simulink model "sl_RobotReal_RRR"  (R2018a)
settings: Solver=ode45  StartTime=0.0  StopTime=30  MaxStep=1e-3  RelTol=1e-3  EnableMultiTasking=on
values from neighbouring files (symbols this model uses):
  Aa_1 = Aa_1/50    (= 0.004)    [DatosSimAcDir_Exp.m]    (also in DatosSimSenoides.m = 1; DatosSimSenoides_Exp.m = 2)
  Aa_2 = Aa_2/30    (= 6.66666666667)    [DatosSimAcDir_Exp.m]    (also in DatosSimSenoides.m = 1; DatosSimSenoides_Exp.m = 0.5)
  Aa_3 = Aa_3/15    (= 0.266666666667)    [DatosSimAcDir_Exp.m]    (also in DatosSimSenoides.m = 5; DatosSimSenoides_Exp.m = 0.5)
  Ab_1 = Ab_1/50    (= 6e-05)    [DatosSimAcDir_Exp.m]    (also in DatosSimSenoides.m = 2; DatosSimSenoides_Exp.m = 3)
  Ab_3 = Ab_3/15    (= 1)    [DatosSimAcDir_Exp.m]    (also in DatosSimSenoides.m = 6; DatosSimSenoides_Exp.m = 2)
  Im_cc1 = Im_cc1/50    (= 0)    [DatosSimAcDir_Exp.m]    (also in DatosSimSenoides.m; DatosSimSenoides_Exp.m)
  Im_cc2 = Im_cc2/30    (= 96.6666666667)    [DatosSimAcDir_Exp.m]    (also in DatosSimSenoides.m = 0; DatosSimSenoides_Exp.m = 14)
  Im_cc3 = Im_cc3/15    (= 1)    [DatosSimAcDir_Exp.m]    (also in DatosSimSenoides.m = 0; DatosSimSenoides_Exp.m = 3)
  R1 = 50    [AnalisisFrecuencial.m]    (also in ComparativaModelo.m; DinamicaNE_RRR.m = R1; IdentificacParamDinam.m; Modelado_Dinamico_Gs.m = 1)
  R2 = 30    [AnalisisFrecuencial.m]    (also in ComparativaModelo.m; DinamicaNE_RRR.m = R2; IdentificacParamDinam.m; Modelado_Dinamico_Gs.m = 1)
  R3 = 15    [AnalisisFrecuencial.m]    (also in ComparativaModelo.m; DinamicaNE_RRR.m = R3; IdentificacParamDinam.m; Modelado_Dinamico_Gs.m = 1)
  tau1 = 1    [DatosSimAcDir_Exp.m]    (also in DatosSimSenoides.m = 5; DatosSimSenoides_Exp.m = 0.01)
  tau2 = 100    [DatosSimAcDir_Exp.m]    (also in DatosSimSenoides.m = 5; DatosSimSenoides_Exp.m = 1)
  tau3 = 20    [DatosSimAcDir_Exp.m]    (also in DatosSimSenoides.m = 5; DatosSimSenoides_Exp.m = 0.01)
  Tm = 0.001    [AnalisisFrecuencial.m]    (also in ComparativaModelo.m; DatosSimSenoides.m = 0.01; GDT_C_RRR.m; controlador.m)
  wa_1 = 10    [DatosSimAcDir_Exp.m]    (also in DatosSimSenoides.m = 0.5; DatosSimSenoides_Exp.m)
  wa_2 = 40    [DatosSimAcDir_Exp.m]    (also in DatosSimSenoides.m = 3; DatosSimSenoides_Exp.m = 15)
  wa_3 = 8    [DatosSimAcDir_Exp.m]    (also in DatosSimSenoides.m = 0.5; DatosSimSenoides_Exp.m)
  wb_1 = 3    [DatosSimAcDir_Exp.m]    (also in DatosSimSenoides.m = 1; DatosSimSenoides_Exp.m)
  wb_3 = 50    [DatosSimAcDir_Exp.m]    (also in DatosSimSenoides.m = 1; DatosSimSenoides_Exp.m = 3)
settings Model: ExtModeTrigMode=oneshot  ExtModeArmWhenConnect=off  Creator=mortega  LastModifiedBy=MAMG
settings DataIOCC: SaveFormat=Array  SignalLoggingSaveFormat=ModelDataLogs
settings OptimizationCC: BlockReduction=off  BooleanDataType=off  ExpressionDepthLimit=2147483647  InitFltsAndDblsToZero=on  LifeSpan=inf
settings DebuggingCC: SaveWithParameterizedLinksMsg=none  UnderspecifiedInitializationDetection=Classic  MergeDetectMultiDrivingBlocksExec=none  SignalResolutionControl=TryResolveAllWithWarning  MultiTaskDSMMsg=warning  MultiTaskCondExecSysMsg=none  FcnCallInpInsideContextMsg=warning  StateNameClashWarn=warning  SFUnexpectedBacktrackingDiag=warning  SFNoUnconditionalDefaultTransitionDiag=warning  SFExecutionAtInitializationDiag=none
settings HardwareCC: ProdBitPerPointer=32  ProdBitPerSizeT=32  ProdBitPerPtrDiffT=32  ProdLargestAtomicFloat=None  ProdIntDivRoundTo=Undefined  ProdEndianess=Unspecified  ProdWordSize=32  ProdHWDeviceType=32-bit Generic  TargetUnknown=on
settings ModelReferenceCC: PropagateSignalLabelsOutOfModel=off
settings CodeAppCC: StateflowObjectComments=on
settings GRTTargetCC: TargetFcnLib=ansi_tfl_tmw.mat  TargetLangStandard=C89/C90 (ANSI)  CombineOutputUpdateFcns=off  GRTInterface=on
settings ConfigComp: CovMetricSettings=dw  CovHtmlReporting=on  CovSaveCumulativeToWorkspaceVar=on  CovSaveSingleToWorkspaceVar=on  CovExternalEMLEnable=off

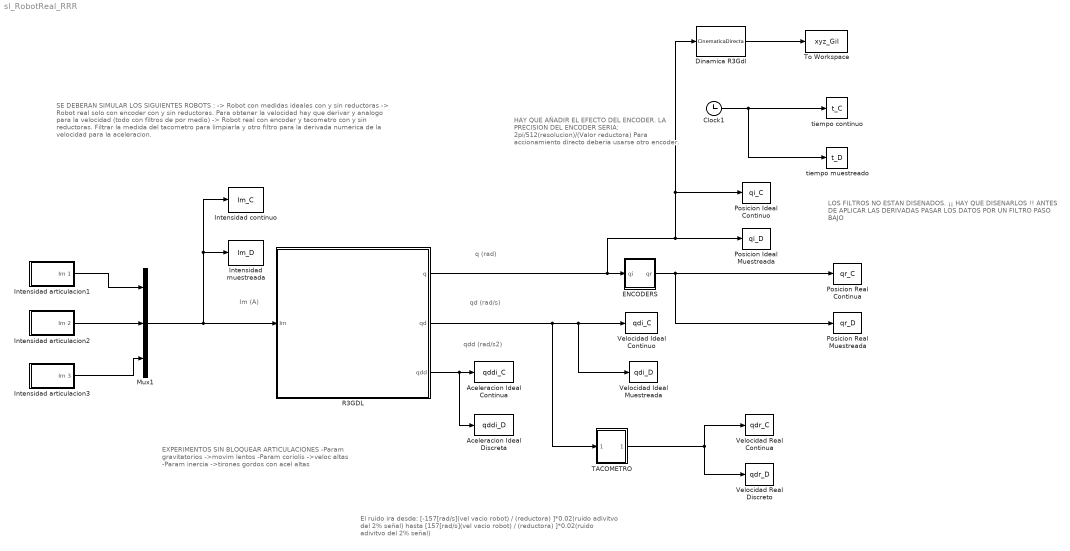
== system sl_RobotReal_RRR ==
  note: LOS FILTROS NO ESTAN DISENADOS.
      | ¡¡ HAY QUE DISENARLOS !!
      |
      | ANTES DE APLICAR LAS DERIVADAS PASAR
      | LOS DATOS POR UN FILTRO PASO BAJO
  note: SE DEBERAN SIMULAR LOS SIGUIENTES ROBOTS :
      | -> Robot con medidas ideales con y sin reductoras
      | -> Robot real solo con encoder con y sin reductoras. Para obtener la velocidad hay que derivar
      | y analogo para la velocidad
      | (todo con filtros de por medio)
      | -> Robot real con encoder y tacometro con y sin reductoras. Filtrar la medida del tacometro para limpiarla
      | y otro filtro para la derivada numerica de la
      | velocidad para la aceleracion.
  note: EXPERIMENTOS SIN BLOQUEAR ARTICULACIONES
      | -Param gravitatorios ->movim lentos
      | -Param coriolis ->veloc altas
      | -Param inercia ->tirones gordos con acel altas
  note: El ruido ira desde:
      | [-157[rad/s](vel vacio robot) / (reductora) ]*0.02(ruido adivitvo del 2% señal)
      | hasta
      | [157[rad/s](vel vacio robot) / (reductora) ]*0.02(ruido adivitvo del 2% señal)
  note: HAY QUE AÑADIR EL EFECTO DEL ENCODER.
      | LA PRECISION DEL ENCODER SERIA:
      | 2pi/512(resolucion)/(Valor reductora)
      |
      | Para accionamiento directo deberia usarse otro
      | encoder.
  note: Im (A)
  note: q (rad)
  note: qd (rad/s)
  note: qdd (rad/s2)
  Aceleracion Ideal Continua : ToWorkspace  VariableName=qddi_C  SampleTime=-1
  Aceleracion Ideal Discreta : ToWorkspace  VariableName=qddi_D  SampleTime=Tm
  Clock1 : Clock
  Dinamica R3Gdl : MATLABFcn  MATLABFcn=CinematicaDirecta  OutputDimensions=3
  ENCODERS : Subsystem
  Intensidad continuo : ToWorkspace  VariableName=Im_C  SampleTime=-1
  Intensidad articulacion1 : Subsystem
  Intensidad articulacion2 : Subsystem
  Intensidad articulacion3 : Subsystem
  "Intensidad muestreada " : ToWorkspace  VariableName=Im_D  SampleTime=Tm
  Mux1 : Mux  Inputs=3
  Posicion Ideal Continuo : ToWorkspace  VariableName=qi_C  SampleTime=-1
  Posicion Ideal Muestreada : ToWorkspace  VariableName=qi_D  SampleTime=Tm
  Posicion Real Continua : ToWorkspace  VariableName=qr_C  SampleTime=-1
  Posicion Real Muestreada : ToWorkspace  VariableName=qr_D  SampleTime=Tm
  R3GDL : Subsystem  mask(Control y Programación de Robots (4 GIERM)){NGrupo=11, q1_ini=0, q2_ini=-pi/4, q3_ini=0, Bl_q1=off, Bl_q2=off, Bl_q3=off, AccionamientoDirecto=off}
      mask prompts: NGrupo "Nº de GRUPO"; q1_ini "q1 inicial  (rad)"; q2_ini "q2 inicial (rad)"; q3_ini "q3_inicial (rad)"; Bl_q1 "Bloqueo q1"; Bl_q2 "Bloqueo q2"; Bl_q3 "Bloqueo q3"; AccionamientoDirecto "Accionamiento directo"
      mask help: Robot de 3 grados de libertad RRR
      mask Display:
      | image(imread('R3GDL_RRR.JPG'));
      | port_label('output', 1, 'q');
      | port_label('output', 2, 'qd');
      | port_label('output', 3, 'qdd');
      | port_label('input', 1, 'Im')
  TACOMETRO : Subsystem
  To Workspace : ToWorkspace  VariableName=xyz_Gil  SampleTime=Tm
  Velocidad Ideal Continuo : ToWorkspace  VariableName=qdi_C  SampleTime=-1
  Velocidad Ideal Muestreada : ToWorkspace  VariableName=qdi_D  SampleTime=Tm
  Velocidad Real Continua : ToWorkspace  VariableName=qdr_C  SampleTime=-1
  Velocidad Real Discreto : ToWorkspace  VariableName=qdr_D  SampleTime=Tm
  tiempo muestreado : ToWorkspace  VariableName=t_D  SampleTime=Tm
  tiempo continuo : ToWorkspace  VariableName=t_C  SampleTime=-1
  wires:
  TACOMETRO/1(qdr) -> Velocidad Real Continua/1, Velocidad Real Discreto/1
  Clock1/1 -> tiempo continuo/1, tiempo muestreado/1
  R3GDL/2(qd) -> TACOMETRO/1(qdi), Velocidad Ideal Muestreada/1, Velocidad Ideal Continuo/1
  R3GDL/3(qdd) -> Aceleracion Ideal Continua/1, Aceleracion Ideal Discreta/1
  Mux1/1 -> "Intensidad muestreada "/1, Intensidad continuo/1, R3GDL/1(Im)
  ENCODERS/1(qr) -> Posicion Real Continua/1, Posicion Real Muestreada/1
  R3GDL/1(q) -> Dinamica R3Gdl/1, Posicion Ideal Continuo/1, Posicion Ideal Muestreada/1, ENCODERS/1(qi)
  Dinamica R3Gdl/1 -> To Workspace/1
  Intensidad articulacion1/1(Im 1) -> Mux1/1
  Intensidad articulacion3/1(Im 3) -> Mux1/3
  Intensidad articulacion2/1(Im 2) -> Mux1/2

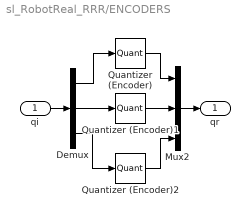
== system sl_RobotReal_RRR/ENCODERS ==
  qi : Inport
  Demux : Demux  Outputs=3
  Mux2 : Mux  Inputs=3
  Quantizer (Encoder) : Quantizer  QuantizationInterval=2*pi/512/R1
  Quantizer (Encoder)1 : Quantizer  QuantizationInterval=2*pi/512/R2
  Quantizer (Encoder)2 : Quantizer  QuantizationInterval=2*pi/512/R3
  qr : Outport
  wires:
  Demux/2 -> Quantizer (Encoder)1/1
  Demux/1 -> Quantizer (Encoder)/1
  Quantizer (Encoder)1/1 -> Mux2/2
  Mux2/1 -> qr/1
  Quantizer (Encoder)2/1 -> Mux2/3
  Demux/3 -> Quantizer (Encoder)2/1
  qi/1 -> Demux/1
  Quantizer (Encoder)/1 -> Mux2/1

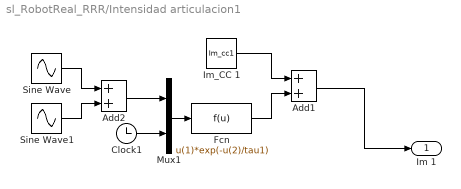
== system sl_RobotReal_RRR/Intensidad articulacion1 ==
  Add1 : Sum
  Add2 : Sum
  Clock1 : Clock
  Fcn : Fcn  Expr=u(1)*exp(-u(2)/tau1)
  "Im_CC 1 " : Constant  Value=Im_cc1
  Mux1 : Mux  Inputs=2
  Sine Wave : Sin  Amplitude=Aa_1  Frequency=wa_1  SampleTime=0
  Sine Wave1 : Sin  Amplitude=Ab_1  Frequency=wb_1  SampleTime=0
  Im 1 : Outport
  wires:
  Add2/1 -> Mux1/1
  "Im_CC 1 "/1 -> Add1/1
  Fcn/1 -> Add1/2
  Clock1/1 -> Mux1/2
  Add1/1 -> Im 1/1
  Mux1/1 -> Fcn/1
  Sine Wave1/1 -> Add2/2
  Sine Wave/1 -> Add2/1

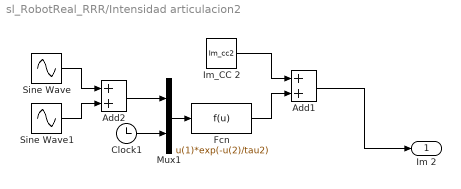
== system sl_RobotReal_RRR/Intensidad articulacion2 ==
  Add1 : Sum
  Add2 : Sum
  Clock1 : Clock
  Fcn : Fcn  Expr=u(1)*exp(-u(2)/tau2)
  "Im_CC 2 " : Constant  Value=Im_cc2
  Mux1 : Mux  Inputs=2
  Sine Wave : Sin  Amplitude=Aa_2  Frequency=wa_2  SampleTime=0
  Sine Wave1 : Sin  Amplitude=Ab_1  Frequency=wb_1  SampleTime=0
  Im 2 : Outport
  wires:
  Add2/1 -> Mux1/1
  "Im_CC 2 "/1 -> Add1/1
  Fcn/1 -> Add1/2
  Clock1/1 -> Mux1/2
  Add1/1 -> Im 2/1
  Mux1/1 -> Fcn/1
  Sine Wave1/1 -> Add2/2
  Sine Wave/1 -> Add2/1

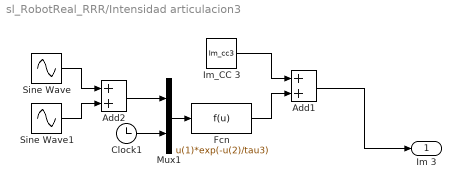
== system sl_RobotReal_RRR/Intensidad articulacion3 ==
  Add1 : Sum
  Add2 : Sum
  Clock1 : Clock
  Fcn : Fcn  Expr=u(1)*exp(-u(2)/tau3)
  "Im_CC 3 " : Constant  Value=Im_cc3
  Mux1 : Mux  Inputs=2
  Sine Wave : Sin  Amplitude=Aa_3  Frequency=wa_3  SampleTime=0
  Sine Wave1 : Sin  Amplitude=Ab_3  Frequency=wb_3  SampleTime=0
  Im 3 : Outport
  wires:
  Add2/1 -> Mux1/1
  "Im_CC 3 "/1 -> Add1/1
  Fcn/1 -> Add1/2
  Clock1/1 -> Mux1/2
  Add1/1 -> Im 3/1
  Mux1/1 -> Fcn/1
  Sine Wave1/1 -> Add2/2
  Sine Wave/1 -> Add2/1

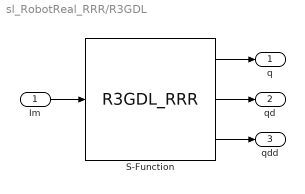
== system sl_RobotReal_RRR/R3GDL ==
  Im : Inport
  S-Function : S-Function  FunctionName=R3GDL_RRR  Parameters=[q1_ini; q2_ini; q3_ini]; [Bl_q1; Bl_q2; Bl_q3]; AccionamientoDirecto; NGrupo  SFunctionDeploymentMode=off  EnableBusSupport=off
  q : Outport
  qd : Outport  Port=2
  qdd : Outport  Port=3
  wires:
  Im/1 -> S-Function/1
  S-Function/1 -> q/1
  S-Function/2 -> qd/1
  S-Function/3 -> qdd/1

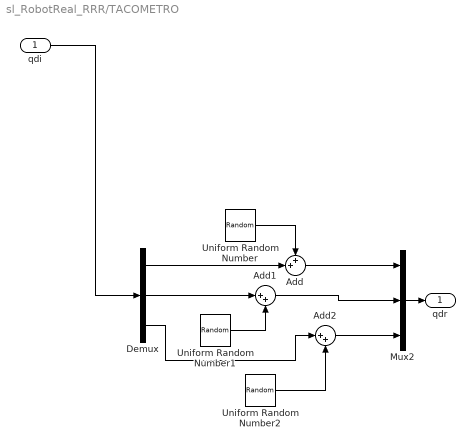
== system sl_RobotReal_RRR/TACOMETRO ==
  qdi : Inport
  Add : Sum  Inputs=++|
  Add1 : Sum  Inputs=|++
  Add2 : Sum  Inputs=|++
  Demux : Demux  Outputs=3
  Mux2 : Mux  Inputs=3
  Uniform Random Number : UniformRandomNumber  Minimum=-(157/R1)*0.02  Maximum=(157/R1)*0.02  SampleTime=Tm
  Uniform Random Number1 : UniformRandomNumber  Minimum=-(157/R2)*0.02  Maximum=(157/R2)*0.02  SampleTime=Tm
  Uniform Random Number2 : UniformRandomNumber  Minimum=-(157/R3)*0.02  Maximum=(157/R3)*0.02  SampleTime=Tm
  qdr : Outport
  wires:
  Demux/2 -> Add1/1
  Add1/1 -> Mux2/2
  Add/1 -> Mux2/1
  Demux/1 -> Add/2
  Uniform Random Number1/1 -> Add1/2
  Add2/1 -> Mux2/3
  Uniform Random Number2/1 -> Add2/2
  Uniform Random Number/1 -> Add/1
  Demux/3 -> Add2/1
  Mux2/1 -> qdr/1
  qdi/1 -> Demux/1
